simulink model "sedemo_server_service_time"  (Simulink 7.5)
settings: Solver=VariableStepDiscrete  StartTime=0.0  StopTime=10.0  MaxStep=inf  RelTol=1e-3
libraries: simeventssink1 x9, simeventsgenerators1 x7, simeventsserver1 x3, simeventsinfo x1, simeventsattributes2 x1
settings Model: Creator=The MathWorks Inc.  ExtModeAutoUpdateStatusClock=off
settings DataIOCC: SaveOutput=off  SignalLogging=off  SaveTime=off
settings OptimizationCC: InitFltsAndDblsToZero=on
settings DebuggingCC: AlgebraicLoopMsg=error  SignalResolutionControl=TryResolveAllWithWarning  SolverPrmCheckMsg=none  MultiTaskDSMMsg=warning  MultiTaskCondExecSysMsg=none  SigSpecEnsureSampleTimeMsg=none  StrictBusMsg=None
settings RTWCC: IncludeERTFirstTime=on
settings SimEventsCC: propIdentEventSeed=12345678  propDiagAttribOutput=1  propDiagFcnCallOutput=1  propDiagStatOutput=0

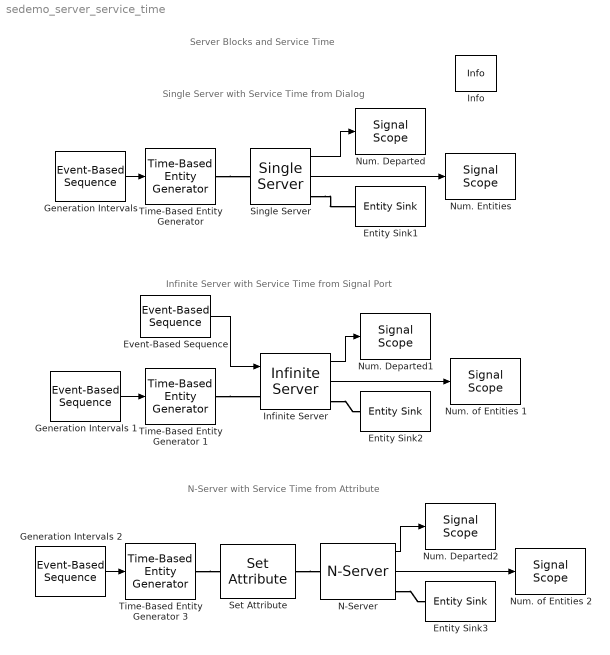
== system sedemo_server_service_time ==
  note: Server Blocks and Service Time
  note: Single Server with Service Time from Dialog
  note: Infinite Server with Service Time from Signal Port
  note: N-Server with Service Time from Attribute
  Entity Sink1 : simeventssink1/Entity Sink  Priority=1  SystemSampleTime=-1  AvailableForArrivals=on  StatNumberArrived=Off
  Entity Sink2 : simeventssink1/Entity Sink  Priority=1  SystemSampleTime=-1  AvailableForArrivals=on  StatNumberArrived=Off
  Entity Sink3 : simeventssink1/Entity Sink  Priority=1  SystemSampleTime=-1  AvailableForArrivals=on  StatNumberArrived=Off
  Event-Based Sequence : simeventsgenerators1/Signal Generators/Event-Based Sequence  SystemSampleTime=-1  VectorOutputValues=[1 1.5 2].'  FormOutputOpt=Cyclic repetition  IsProcessed=on  isConnected=1
  Generation Intervals : simeventsgenerators1/Signal Generators/Event-Based Sequence  SystemSampleTime=-1  VectorOutputValues=[1 2 1 .5 .3 .1].'  FormOutputOpt=Cyclic repetition  IsProcessed=on  isConnected=1
  Generation Intervals 1 : simeventsgenerators1/Signal Generators/Event-Based Sequence  SystemSampleTime=-1  VectorOutputValues=[1 2 1 .5 .3 .1].'  FormOutputOpt=Cyclic repetition  IsProcessed=on  isConnected=1
  Generation Intervals 2 : simeventsgenerators1/Signal Generators/Event-Based Sequence  SystemSampleTime=-1  VectorOutputValues=[1 2 1 .5 .3 .1].'  FormOutputOpt=Cyclic repetition  IsProcessed=on  isConnected=1
  Infinite Server : simeventsserver1/Infinite Server  Priority=1  SystemSampleTime=-1  ServiceTimeFrom=Signal port t  ServiceTime=1.5  AttributeName=myDelayTime  PriorityServiceCompletion=300  EnableTOPort=off  StatNumberDeparted=On  StatNumberInBlock=On  StatPendingEntity=Off  StatNumberPending=Off  StatAverageWait=Off  StatNumberTimedout=Off
  Info : simeventsinfo/Info  SystemSampleTime=-1
  N-Server : simeventsserver1/N-Server  Priority=1  SystemSampleTime=-1  NumberOfServers=3  ServiceTimeFrom=Attribute  ServiceTime=1  AttributeName=myServiceTime  PriorityServiceCompletion=500  EnableTOPort=off  StatNumberDeparted=On  StatNumberInBlock=On  StatPendingEntity=Off  StatNumberPending=Off  StatAverageWait=Off  StatUtilization=Off  StatNumberTimedout=Off
  Num. Departed : simeventssink1/Signal Scope  Priority=1  SystemSampleTime=-1  PlotType=Stair  InputType=Signal  NumInputs=1  AttributeNameY=Count  XInputOptionSignal=Event time  XInputOptionEntity=Event time  AttributeNameX=Count  EnableEntityOutport=on  XMin=0  XMax=10  XLimitExceededOption=Stretch axis limits  YLimitExceededOption=Stretch axis limits  AxisGrid=on  AxisLegend=off  LineDisables=""  LineColors=b  LineStyles=-  LineMarkers=.  OpenScopeAtSimStart=on  Title=Number of Entities Departed Single Server  YLabel=Number of Entities  XLabel=Time  FigurePosition=[636 721 283 129]  AxisZoom=off  DataStoreOption=Limited  DataPointsLimit=10000  StatNumberArrived=Off  ShowCountPlotted=off  ShowToolbar=on
      settings: YMin=0  YMax=10
  Num. Departed1 : simeventssink1/Signal Scope  Priority=1  SystemSampleTime=-1  PlotType=Stair  InputType=Signal  NumInputs=1  AttributeNameY=Count  XInputOptionSignal=Event time  XInputOptionEntity=Event time  AttributeNameX=Count  EnableEntityOutport=on  XMin=0  XMax=10  XLimitExceededOption=Stretch axis limits  YLimitExceededOption=Stretch axis limits  AxisGrid=on  AxisLegend=off  LineDisables=""  LineColors=b  LineStyles=-  LineMarkers=.  OpenScopeAtSimStart=on  Title=Number of Entities Departed Infinite Server  YLabel=Number of Entities  XLabel=Time  FigurePosition=[637 506 281 130]  AxisZoom=off  DataStoreOption=Limited  DataPointsLimit=10000  StatNumberArrived=Off  ShowCountPlotted=off  ShowToolbar=on
      settings: YMin=0  YMax=10
  Num. Departed2 : simeventssink1/Signal Scope  Priority=1  SystemSampleTime=-1  PlotType=Stair  InputType=Signal  NumInputs=1  AttributeNameY=Count  XInputOptionSignal=Event time  XInputOptionEntity=Event time  AttributeNameX=Count  EnableEntityOutport=on  XMin=0  XMax=10  XLimitExceededOption=Stretch axis limits  YLimitExceededOption=Stretch axis limits  AxisGrid=on  AxisLegend=off  LineDisables=""  LineColors=b  LineStyles=-  LineMarkers=.  OpenScopeAtSimStart=on  Title=Number of Entities Departed N-Server  YLabel=Number of Entities  XLabel=Time  FigurePosition=[638 291 282 127]  AxisZoom=off  DataStoreOption=Limited  DataPointsLimit=10000  StatNumberArrived=Off  ShowCountPlotted=off  ShowToolbar=on
      settings: YMin=0  YMax=10
  "Num. Entities " : simeventssink1/Signal Scope  Priority=1  SystemSampleTime=-1  PlotType=Stair  InputType=Signal  NumInputs=1  AttributeNameY=Count  XInputOptionSignal=Event time  XInputOptionEntity=Event time  AttributeNameX=Count  EnableEntityOutport=on  XMin=0  XMax=10  XLimitExceededOption=Stretch axis limits  YLimitExceededOption=Stretch axis limits  AxisGrid=on  AxisLegend=off  LineDisables=""  LineColors=b  LineStyles=-  LineMarkers=.  OpenScopeAtSimStart=on  Title=Number of Entities in Single Server  YLabel=Number of Entities  XLabel=Time  FigurePosition=[367 722 260 130]  AxisZoom=off  DataStoreOption=Limited  DataPointsLimit=10000  StatNumberArrived=Off  ShowCountPlotted=off  ShowToolbar=on
      settings: YMin=0  YMax=5
  Num. of Entities 1 : simeventssink1/Signal Scope  Priority=1  SystemSampleTime=-1  PlotType=Stair  InputType=Signal  NumInputs=1  AttributeNameY=Count  XInputOptionSignal=Event time  XInputOptionEntity=Event time  AttributeNameX=Count  EnableEntityOutport=on  XMin=0  XMax=10  XLimitExceededOption=Stretch axis limits  YLimitExceededOption=Stretch axis limits  AxisGrid=on  AxisLegend=off  LineDisables=""  LineColors=b  LineStyles=-  LineMarkers=.  OpenScopeAtSimStart=on  Title=Number of Entities in Infinite Server  YLabel=Number of Entities  XLabel=Time  FigurePosition=[369 506 260 130]  AxisZoom=off  DataStoreOption=Limited  DataPointsLimit=10000  StatNumberArrived=Off  ShowCountPlotted=off  ShowToolbar=on
      settings: YMin=0  YMax=5
  Num. of Entities 2 : simeventssink1/Signal Scope  Priority=1  SystemSampleTime=-1  PlotType=Stair  InputType=Signal  NumInputs=1  AttributeNameY=Count  XInputOptionSignal=Event time  XInputOptionEntity=Event time  AttributeNameX=Count  EnableEntityOutport=on  XMin=0  XMax=10  XLimitExceededOption=Stretch axis limits  YLimitExceededOption=Stretch axis limits  AxisGrid=on  AxisLegend=off  LineDisables=""  LineColors=b  LineStyles=-  LineMarkers=.  OpenScopeAtSimStart=on  Title=Number of Entities in N-Server  YLabel=Number of Entities  XLabel=Time  FigurePosition=[368 288 260 130]  AxisZoom=off  DataStoreOption=Limited  DataPointsLimit=10000  StatNumberArrived=Off  ShowCountPlotted=off  ShowToolbar=on
      settings: YMin=0  YMax=5
  Set Attribute : simeventsattributes2/Set Attribute  Priority=1  DialogController=des_ddg_create  DialogControllerArgs=DataTag12  SystemSampleTime=-1  AttributeFrom=Dialog  AttributeName=myServiceTime  AttributeTreatAsVector=1  AttributeValue=1.5  AttributeCreate=on  StatNumberDeparted=Off  EvaluatedAttributeValue={1.5}
  Single Server : simeventsserver1/Single Server  Priority=1  SystemSampleTime=-1  ServiceTimeFrom=Dialog  ServiceTime=1  AttributeName=ServiceTime  PriorityServiceCompletion=500  PermitPreemption=off  SortingAttributeName=PriorityAttributeName  SortingDirection=Ascending  WriteToAttribute=off  ResidualAttributeName=ResidualServiceTime  CreateAttribute=on  EnableTOPort=off  StatNumberDeparted=On  StatNumberInBlock=On  StatNumberPreempted=Off  StatPendingEntity=Off  StatAverageWait=Off  StatUtilization=Off  StatNumberTimedout=Off
  Time-Based Entity Generator : simeventsgenerators1/Entity Generators/Time-Based Entity Generator  Priority=1  DialogController=des_ddg_create  DialogControllerArgs=DataTag15  SystemSampleTime=-1  GenerateEntitiesUpon=Intergeneration time from port t  Distribution=Uniform  Minimum=1  Maximum=2  Mean=1  InitialSeed=12345  Period=1  PriorityEntityGeneration=500  GenerateEntityAtSimulationStart=on  ResponseWhenBlocked=Pause generation  ResponseWhenUnblocked=Immediate restart  EntityType=Standard  StatNumberDeparted=Off  StatPendingEntity=Off  StatAverageIntergenerationTime=Off
  Time-Based Entity Generator 1 : simeventsgenerators1/Entity Generators/Time-Based Entity Generator  Priority=1  DialogController=des_ddg_create  DialogControllerArgs=DataTag17  SystemSampleTime=-1  GenerateEntitiesUpon=Intergeneration time from port t  Distribution=Uniform  Minimum=1  Maximum=2  Mean=1  InitialSeed=12345  Period=1  PriorityEntityGeneration=500  GenerateEntityAtSimulationStart=on  ResponseWhenBlocked=Pause generation  ResponseWhenUnblocked=Immediate restart  EntityType=Standard  StatNumberDeparted=Off  StatPendingEntity=Off  StatAverageIntergenerationTime=Off
  Time-Based Entity Generator 3 : simeventsgenerators1/Entity Generators/Time-Based Entity Generator  Priority=1  DialogController=des_ddg_create  DialogControllerArgs=DataTag19  SystemSampleTime=-1  GenerateEntitiesUpon=Intergeneration time from port t  Distribution=Uniform  Minimum=1  Maximum=2  Mean=1  InitialSeed=12345  Period=1  PriorityEntityGeneration=500  GenerateEntityAtSimulationStart=on  ResponseWhenBlocked=Pause generation  ResponseWhenUnblocked=Immediate restart  EntityType=Standard  StatNumberDeparted=Off  StatPendingEntity=Off  StatAverageIntergenerationTime=Off
  wires:
  Single Server/1 -> Num. Departed/1
  Generation Intervals/1 -> Time-Based Entity Generator/1
  Single Server/2 -> "Num. Entities "/1
  Infinite Server/1 -> Num. Departed1/1
  Generation Intervals 1/1 -> Time-Based Entity Generator 1/1
  Infinite Server/2 -> Num. of Entities 1/1
  Event-Based Sequence/1 -> Infinite Server/1
  N-Server/1 -> Num. Departed2/1
  Generation Intervals 2/1 -> Time-Based Entity Generator 3/1
  N-Server/2 -> Num. of Entities 2/1
  connections:
  Single Server/RConn1 -- Entity Sink1/LConn1
  Time-Based Entity Generator/RConn1 -- Single Server/LConn1
  Infinite Server/RConn1 -- Entity Sink2/LConn1
  Time-Based Entity Generator 1/RConn1 -- Infinite Server/LConn1
  N-Server/RConn1 -- Entity Sink3/LConn1
  Time-Based Entity Generator 3/RConn1 -- Set Attribute/LConn1
  Set Attribute/RConn1 -- N-Server/LConn1
